simulink model "slabo3"  (R2018a)
settings: Solver=FixedStepAuto  StartTime=0.0  StopTime=10.0  FixedStep=0.0001  RelTol=1e-3
values from neighbouring files (symbols this model uses):
  dfc = poly([pcr1;pcr2])    [labo3.m]
  dH = conv([1 0], [1,0.5])    [labo3-nous.m]    (also in labo3.m = conv([1 0],[1 0.5]))
  h = 0.1    [labo3-nous.m]    (also in labo3.m)
  nfc = dfc(3)    [labo3.m]
  nH = 1    [labo3-nous.m]    (also in labo3.m)
undefined symbols (not defined in the file or in its folder): df, dzd, nf, nzd
settings Model: Creator=armenhagopian  LastModifiedBy=alexis
settings CodeAppCC: StateflowObjectComments=on

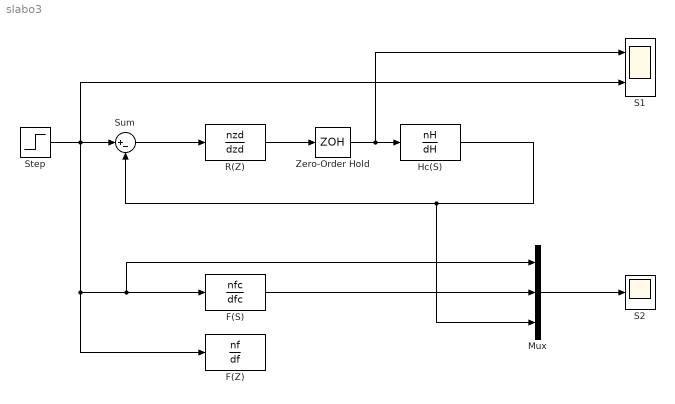
== system slabo3 ==
  F(S) : TransferFcn  Numerator=nfc  Denominator=dfc
  F(Z) : DiscreteTransferFcn  Numerator=nf  Denominator=df  SampleTime=h
  Hc(S) : TransferFcn  Numerator=nH  Denominator=dH
  Mux : Mux  Inputs=3
  R(Z) : DiscreteTransferFcn  Numerator=nzd  Denominator=dzd  SampleTime=h
  S1 : Scope  NumInputPorts=2
  S2 : Scope
  Step : Step  Time=0.5
  Sum : Sum  Inputs=|+-
  Zero-Order Hold : ZeroOrderHold  SampleTime=-1
  wires:
  Sum/1 -> R(Z)/1
  R(Z)/1 -> Zero-Order Hold/1
  Zero-Order Hold/1 -> S1/1, Hc(S)/1
  Hc(S)/1 -> Mux/3, Sum/2
  F(S)/1 -> Mux/2
  Mux/1 -> S2/1
  Step/1 -> S1/2, F(Z)/1, F(S)/1, Mux/1, Sum/1
